simulink model "APE_Project_Closed Loop With Battery_SOC"  (R2025a)
settings: Solver=VariableStepAuto  StartTime=0.0  StopTime=0.05  RelTol=1e-3
undefined symbols (not defined in the file): Ion, Lithium
libraries: spsPWMGeneratorDCDCLib x8, spsCurrentMeasurementLib x5, spsMosfetLib x4, spsSeriesRLCBranchLib x4, spsVoltageMeasurementLib x3, spsBatteryLib x1, spsDCVoltageSourceLib x1, spsDiodeLib x1, spsGroundLib x1, eeStairGenerator x1, sps_lib x1
settings Model: Creator=KAILASH  LastModifiedBy=KAILASH

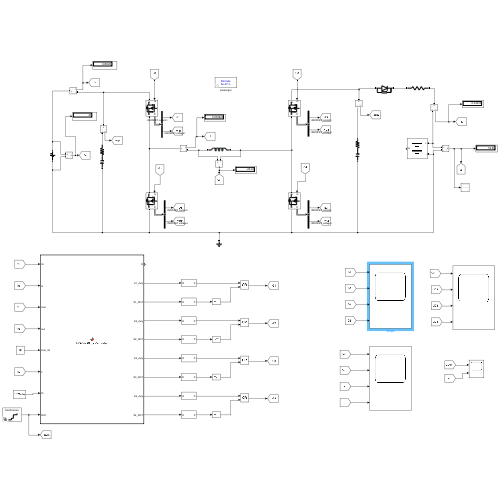
[thumbnail: Simulink's stored preview of the top-level diagram]
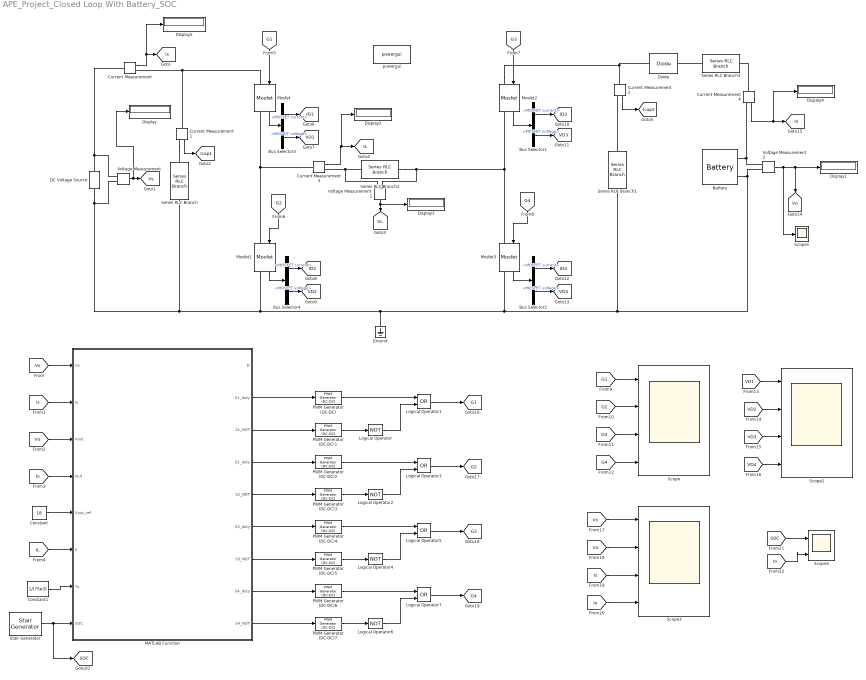
== system APE_Project_Closed Loop With Battery_SOC ==
  Battery : spsBatteryLib/Battery  BatType=Lithium-Ion  NomV=18  NomQ=5.4  SOC=95  Batt_Tr=30  PresetModel=on  MaxQ=5.4  MinV=13.5  FullV=20.9518  Dis_rate=2.3478  R=0.033333  Normal_OP=4.8835  expZone="[19.4469     0.265304]"
  Bus Selector{1..4} (4 alike) : BusSelector  OutputSignals=MOSFET current,MOSFET voltage
  Constant : Constant  Value=18
  Constant1 : Constant  Value=1/(75e3)
  Current Measurement{,1..4} (5 alike) : spsCurrentMeasurementLib/Current Measurement  PhasorSimulation=off  OutputType=Complex  PSBequivalent=0
  DC Voltage Source : spsDCVoltageSourceLib/DC Voltage Source  Amplitude=48  Measurements=Voltage
  Diode : spsDiodeLib/Diode  Ron=0.001  Lon=0  Vf=0.8  IC=0  UseSnubber=0  Rs=500  Cs=250e-9  Measurements=off
  Display{,1..5} (6 alike) : Display
  Ground : spsGroundLib/Ground  LConnTagsString=a
  Logical Operator{,2,4,6} (4 alike) : Logic  Operator=NOT  AllPortsSameDT=off  OutDataTypeStr=boolean
  Logical Operator{1,3,5,7} (4 alike) : Logic  Operator=OR  AllPortsSameDT=off  OutDataTypeStr=boolean
  MATLAB Function : MATLAB Function  TreatAsAtomicUnit=on
  Mosfet{,1..3} (4 alike) : spsMosfetLib/Mosfet  Ron=0.01  Lon=0  Rd=0.01  Vfd=0.8  IC=0  Rs=1e5  Cs=inf  Measurements=on
  PWM Generator (DC-DC){,1..7} (8 alike) : spsPWMGeneratorDCDCLib/PWM Generator (DC-DC)  Fsw=75e3  Ts=0
  Scope : Scope  NumInputPorts=4
      settings: ActiveDisplayYMinimum=-0.12499999999999997  ActiveDisplayYMaximum=1.125
  Scope1 : Scope
      settings: ActiveDisplayYMinimum=-2.5104550941550139  ActiveDisplayYMaximum=22.594095847395128
  Scope2 : Scope  NumInputPorts=4
      settings: ActiveDisplayYMinimum=-4.0101855999563254  ActiveDisplayYMaximum=36.044750018114769  DataLoggingVariableName=ScopeData2
  Scope3 : Scope  NumInputPorts=4
      settings: ActiveDisplayYMinimum=38  ActiveDisplayYMaximum=58  DataLoggingVariableName=ScopeData3
  Scope4 : Scope  NumInputPorts=2
      settings: ActiveDisplayYMinimum=10.625000000000002  ActiveDisplayYMaximum=104.375  DataLoggingVariableName=ScopeData4
  Series RLC Branch : spsSeriesRLCBranchLib/Series RLC Branch  LConnTagsString=__new0  RConnTagsString=__new0  BranchType=RC  Resistance=0.001  Inductance=1e-3  SetiL0=off  InitialCurrent=0  Capacitance=488e-6  Setx0=off  InitialVoltage=48  Measurements=None
  Series RLC Branch1 : spsSeriesRLCBranchLib/Series RLC Branch  LConnTagsString=__new0  RConnTagsString=__new0  BranchType=RC  Resistance=0.01  Inductance=1e-3  SetiL0=off  InitialCurrent=0  Capacitance=488e-6  Setx0=off  InitialVoltage=36  Measurements=None
  Series RLC Branch2 : spsSeriesRLCBranchLib/Series RLC Branch  LConnTagsString=__new0  RConnTagsString=__new0  BranchType=L  Resistance=1  Inductance=150e-6  SetiL0=off  InitialCurrent=0  Capacitance=1e-6  Setx0=off  InitialVoltage=0  Measurements=None
  Series RLC Branch3 : spsSeriesRLCBranchLib/Series RLC Branch  LConnTagsString=__new0  RConnTagsString=__new0  BranchType=R  Resistance=1  Inductance=1e-3  SetiL0=off  InitialCurrent=0  Capacitance=1e-6  Setx0=off  InitialVoltage=0  Measurements=None
  Stair Generator : eeStairGenerator/Stair Generator  LabelModeActiveChoice=Continuous  TimeInput=[0 0.02 0.03 0.05]  AmplitudeInput="[20  40 80 95]"  SampleTime=0  RepeatPattern=off  OutDataTypeStr=double
      settings: LibrarySourceBlock=ee_sl_lib/General Control/Stair Generator
  Voltage Measurement : spsVoltageMeasurementLib/Voltage Measurement  PhasorSimulation=off  OutputType=Complex  PSBequivalent=0
  Voltage Measurement1 : spsVoltageMeasurementLib/Voltage Measurement  PhasorSimulation=off  OutputType=Complex  PSBequivalent=0
  Voltage Measurement2 : spsVoltageMeasurementLib/Voltage Measurement  PhasorSimulation=off  OutputType=Complex  PSBequivalent=0
  powergui : sps_lib/powergui  Priority=1  SimulationMode=Discrete  SampleTime=5e-7  frequency=60  Iterations=50  frequencyindice=0  Pbase=100e6  ErrMax=1e-4  UnitsV=kV  UnitsW=MW  buscounter=0  FunctionMessages=off  echomessages=off  EnableUseOfTLC=off  CurrentSourceSwitches=off  DisableSnubberDevices=off  DisableRonSwitches=off  DisableVfSwitches=off  DisplayEquations=off  AutomaticDiscreteSolvers=off  SolverType=Tustin/Backward Euler (TBE)  Interpol=off  ExternalGateDelay=off  methode=off  Ts=100  x0status=blocks  SPID=on  SwTol=0  HookPort=off  NonlinearTolerance=1e-4  nMaxIteration=100  ContinueOnMaxIteration=off  RestoreLinks=warning  ResistiveCurrentMeasurement=off  Frange=[0:2:500]  Ylog=off  Xlog=on  ShowGrid=off  save=off  variable=ZData  structure=0  ZoomFFT=off  StartTime=0.0  cycles=1  DisplayStyle=1  fundamental=60  FreqAxis=off  MaxFrequency=1000  frequencyindicesteady=1  RmsSteady=1  display=off
  tag scope: G1=global, G2=global, G3=global, G4=global, ID1=global, ID2=global, ID3=global, ID4=global, IL=global, Icap1=global, Icap2=global, Io=global, Is=global, SOC=global, VD1=global, VD2=global, VD3=global, VD4=global, VL=global, Vo=global, Vs=global
  wires:
  [G4] -> Mosfet3/1
  Logical Operator3/1 -> [G2]
  [G3] -> Scope/3
  [G1] -> Mosfet/1
  Logical Operator5/1 -> [G3]
  Constant/1 -> MATLAB Function/5(Vout_ref)
  [Vo] -> MATLAB Function/3(Vout)
  MATLAB Function/7(S3_NOT) -> PWM Generator (DC-DC)5/1
  Logical Operator2/1 -> Logical Operator3/2
  PWM Generator (DC-DC)2/1 -> Logical Operator3/1
  PWM Generator (DC-DC)3/1 -> Logical Operator2/1
  [G2] -> Mosfet1/1
  PWM Generator (DC-DC)6/1 -> Logical Operator7/1
  Logical Operator6/1 -> Logical Operator7/2
  [Vs] -> MATLAB Function/1(Vs)
  PWM Generator (DC-DC)7/1 -> Logical Operator6/1
  Logical Operator4/1 -> Logical Operator5/2
  [G1] -> Scope/1
  [G3] -> Mosfet2/1
  [Vo] -> Scope3/2
  Constant1/1 -> MATLAB Function/7(Ts)
  MATLAB Function/6(S3_duty) -> PWM Generator (DC-DC)4/1
  Logical Operator/1 -> Logical Operator1/2
  PWM Generator (DC-DC)1/1 -> Logical Operator/1
  [Is] -> MATLAB Function/2(Is)
  MATLAB Function/8(S4_duty) -> PWM Generator (DC-DC)6/1
  PWM Generator (DC-DC)/1 -> Logical Operator1/1
  Bus Selector1/2 -> [VD3]  "<MOSFET voltage>"
  Current Measurement3/1 -> Display2/1, [IL]
  Current Measurement2/1 -> [Icap2]
  [G2] -> Scope/2
  Bus Selector3/2 -> [VD1]  "<MOSFET voltage>"
  [VD2] -> Scope2/2
  Mosfet1/1 -> Bus Selector4/1
  Bus Selector4/2 -> [VD2]  "<MOSFET voltage>"
  Mosfet/1 -> Bus Selector3/1
  Voltage Measurement1/1 -> Display3/1, [VL]
  Mosfet2/1 -> Bus Selector1/1
  Bus Selector4/1 -> [ID2]  "<MOSFET current>"
  Bus Selector3/1 -> [ID1]  "<MOSFET current>"
  Voltage Measurement/1 -> Display/1, [Vs]
  PWM Generator (DC-DC)4/1 -> Logical Operator5/1
  Logical Operator1/1 -> [G1]
  Current Measurement4/1 -> Display4/1, [Io]
  Voltage Measurement2/1 -> Scope1/1, [Vo], Display1/1
  [VD1] -> Scope2/1
  [VD3] -> Scope2/3
  Current Measurement/1 -> Display5/1, [Is]
  Mosfet3/1 -> Bus Selector2/1
  [IL] -> MATLAB Function/6(Il)
  Logical Operator7/1 -> [G4]
  Bus Selector2/2 -> [VD4]  "<MOSFET voltage>"
  [VD4] -> Scope2/4
  MATLAB Function/5(S2_NOT) -> PWM Generator (DC-DC)3/1
  Bus Selector2/1 -> [ID4]  "<MOSFET current>"
  MATLAB Function/9(S4_NOT) -> PWM Generator (DC-DC)7/1
  [Io] -> Scope3/4
  [Vs] -> Scope3/1
  [G4] -> Scope/4
  [Is] -> Scope3/3
  [Io] -> MATLAB Function/4(Iout)
  PWM Generator (DC-DC)5/1 -> Logical Operator4/1
  Current Measurement1/1 -> [Icap1]
  MATLAB Function/2(S1_duty) -> PWM Generator (DC-DC)/1
  Bus Selector1/1 -> [ID3]  "<MOSFET current>"
  MATLAB Function/4(S2_duty) -> PWM Generator (DC-DC)2/1
  MATLAB Function/3(S1_NOT) -> PWM Generator (DC-DC)1/1
  Stair Generator/1 -> [SOC], MATLAB Function/8(SOC)
  [SOC] -> Scope4/1
  [Io] -> Scope4/2
  connections:
  Mosfet3/LConn1 -- Mosfet2/RConn1 -- Voltage Measurement1/LConn2 -- Series RLC Branch2/RConn1
  Battery/LConn2 -- Voltage Measurement2/LConn2 -- Series RLC Branch1/RConn1 -- Ground/LConn1 -- Mosfet1/RConn1 -- Series RLC Branch/RConn1 -- Voltage Measurement/LConn2 -- DC Voltage Source/LConn1 -- Mosfet3/RConn1
  Mosfet2/LConn1 -- Current Measurement2/LConn1 -- Diode/LConn1
  Voltage Measurement1/LConn1 -- Current Measurement3/RConn1 -- Series RLC Branch2/LConn1
  Battery/LConn1 -- Current Measurement4/RConn1 -- Voltage Measurement2/LConn1
  Voltage Measurement/LConn1 -- Current Measurement/LConn1 -- DC Voltage Source/RConn1
  Current Measurement3/LConn1 -- Mosfet/RConn1 -- Mosfet1/LConn1
  Current Measurement1/LConn1 -- Current Measurement/RConn1 -- Mosfet/LConn1
  Series RLC Branch3/LConn1 -- Diode/RConn1
  Series RLC Branch1/LConn1 -- Current Measurement2/RConn1
  Current Measurement1/RConn1 -- Series RLC Branch/LConn1
  Current Measurement4/LConn1 -- Series RLC Branch3/RConn1

== matlab function APE_Project_Closed Loop With Battery_SOC/MATLAB Function ==
  data: Vs input; D output; Is input; Vout input; Iout input; Vout_ref input; Il input; Ts input; S1_duty output; S1_NOT output; S2_duty output; S2_NOT output; S3_duty output; S3_NOT output; S4_duty output; S4_NOT output; SOC input
function [D, S1_duty, S1_NOT, S2_duty, S2_NOT, S3_duty, S3_NOT, S4_duty, S4_NOT] = biDirBuckBoostController(Vs, Is, Vout, Iout, Vout_ref, Il, Ts, SOC)
% Bidirectional 4-switch DC-DC controller 
% Auto-Mode Detection with Noise-Immune Hysteresis (Deadband)
% Charge Mode: Hybrid SOC Profile + CV Safety Limit
% Discharge Mode: Cascaded Voltage/Current loop with Feedforward
% %#codegen

%% ===================== GLOBAL VARIABLES =====================
% Safety / clamping
D_MAX = 0.92;
D_MIN = 0.1;
V_HYST_CHRG = 4.5; % hysteresis band (V) for topology switching

%% ===================== CHARGING VARIABLES =====================
persistent v_int_chg i_int_chg
if isempty(v_int_chg), v_int_chg = 0; end
if isempty(i_int_chg), i_int_chg = 0; end

% SOC Profile Settings
I_MAX_BULK = 5.0;       % Max current during 0-80% (A)
I_MIN_TAPER = 0.5;      % End-of-charge current at 99% (A)
SOC_BULK_END = 80.0;    % When to start tapering current (%)
SOC_FULL = 100.0;       % When to stop charging completely (%)

% Gains
Kp_v_chg = 0.5;        Ki_v_chg = 15.0;  % Outer CV loop gains (Safety Brake)
Kp_i_chg = 0.05;       Ki_i_chg = 40.0;  % Inner CC loop gains (Muscle)

%% ===================== DISCHARGE VARIABLES =====================
persistent v_int_dis i_int_dis R_est_prev
if isempty(v_int_dis), v_int_dis = 0; end
if isempty(i_int_dis), i_int_dis = 0; end
if isempty(R_est_prev), R_est_prev = 3; end

%% ===================== INITIALIZE OUTPUTS =====================
D = 0.0;
S1_duty = 0.0; S1_NOT  = 1.0;
S2_duty = 0.0; S2_NOT  = 1.0;
S3_duty = 0.0; S3_NOT  = 1.0;
S4_duty = 0.0; S4_NOT  = 1.0;

%% ===================== AUTO MODE DETECTION (DEADBAND) =====================
persistent is_charging_state
if isempty(is_charging_state)
    is_charging_state = true; % Default startup state
end

% The Noise Immunity Band (Amps)
I_DEADBAND = 0.1; 
if is_charging_state == true
    if Il < -I_DEADBAND
        is_charging_state = false;
    end
else
    if Il > I_DEADBAND
        is_charging_state = true;
    end
end
is_charging = is_charging_state;

%% ===================== CHARGE MODE CONTROL (HYBRID SOC) =====================
if is_charging
    
    % --- 1. SOC PROFILE MANAGER ---
    if SOC < SOC_BULK_END
        I_soc_limit = I_MAX_BULK;
    elseif SOC >= SOC_FULL
        I_soc_limit = 0.0;
    else
        % Linear taper down as battery approaches 100%
        fraction = (SOC - SOC_BULK_END) / (SOC_FULL - SOC_BULK_END);
        I_soc_limit = I_MAX_BULK - (fraction * (I_MAX_BULK - I_MIN_TAPER));
    end

    % --- 2. OUTER VOLTAGE LOOP (Safety Brake) ---
    v_err = Vout_ref - Vout;
    v_int_chg = v_int_chg + Ki_v_chg * v_err * Ts;
    
    % Anti-windup: Clamp to the dynamic SOC limit instead of a fixed 5.0A
    v_int_chg = min(max(v_int_chg, 0.0), I_soc_limit);
    
    % Calculate requested current and clamp to dynamic SOC limit
    I_target = Kp_v_chg * v_err + v_int_chg;
    I_target = min(max(I_target, 0.0), I_soc_limit);
    
    % --- 3. INNER CURRENT LOOP ---
    i_err = I_target - Iout;
    i_int_chg = i_int_chg + Ki_i_chg * i_err * Ts;
    i_int_chg = min(max(i_int_chg, D_MIN), D_MAX);
    D_unsat = Kp_i_chg * i_err + i_int_chg;
    
    % Final Saturation & Anti-windup
    if D_unsat > D_MAX
        D = D_MAX;
        i_int_chg = i_int_chg - Ki_i_chg * i_err * Ts;
    elseif D_unsat < D_MIN
        D = D_MIN;
        i_int_chg = i_int_chg - Ki_i_chg * i_err * Ts;
    else
        D = D_unsat;
    end

    % --- SWITCH MAPPING (TOPOLOGY SELECTOR) ---
    if Vs > Vout - V_HYST_CHRG && Vs < Vout + V_HYST_CHRG
        % Buck-boost region
        S1_duty = D;      S1_NOT  = 1.0;
        S2_duty = 0.0;    S2_NOT  = D;
        S3_duty = 0.0;    S3_NOT  = D;
        S4_duty = D;      S4_NOT  = 1.0;
    elseif Vs > Vout + V_HYST_CHRG
        % Buck region
        S1_duty = D;      S1_NOT  = 1.0;
        S2_duty = 0.0;    S2_NOT  = D;
        S3_duty = 1.0;    S3_NOT  = 1.0;
        S4_duty = 0.0;    S4_NOT  = 1.0;
    else
        % Boost region 
        S1_duty = 1.0;    S1_NOT  = 1.0;
        S2_duty = 0.0;    S2_NOT  = 1.0;
        S3_duty = 0.0;    S3_NOT  = D;
        S4_duty = D;      S4_NOT  = 1.0;
    end
    return;

%% ===================== DISCHARGE MODE CONTROL =====================
else
    % ----- Reference & limits -----
    Vref_led      = 14.4;        
    V_HYST_DISCH  = 0.50;        
    I_target_nom  = 1.0;         
    I_abs_max     = 1.4;         
    I_HYST_DISCH  = 0.01;        

    % ----- Gains -----
    Kp_v = 0.12;   Ki_v = 40;   
    Kp_i = 0.45;   Ki_i = 270;  
    FF_mix = 0.6;               

    % ----- Measured variables -----
    I_load = -Is;               
    V_load = Vs;                
    V_batt = Vout;              

    % ================= OUTER VOLTAGE LOOP =================
    v_err = Vref_led - V_load;
    if abs(v_err) > V_HYST_DISCH
        v_int_dis = v_int_dis + Ki_v * v_err * Ts;
    end
    v_int_dis = min(max(v_int_dis, -1.0), 1.0);
    I_target = Kp_v * v_err + v_int_dis + I_target_nom;
    I_target = min(max(I_target, 0.0), I_abs_max);

    % ================= INNER CURRENT LOOP & FEEDFORWARD =================
    epsI = 1e-4;
    R_inst = V_load / max(I_load, epsI);
    alphaR = 0.08;
    R_est = (1 - alphaR) * R_est_prev + alphaR * R_inst;
    R_est_prev = R_est;
    V_load_ff = I_target * R_est;
    if V_load_ff <= V_batt
        D_ff = V_load_ff / max(V_batt, 1e-6);      % buck
    else
        D_ff = 1 - (V_batt / max(V_load_ff, 1e-6)); % boost
    end
    D_ff = min(max(D_ff, D_MIN), D_MAX);

    % Current PI
    i_err = I_target - I_load;
    if abs(i_err) > I_HYST_DISCH
        i_int_dis = i_int_dis + Ki_i * i_err * Ts;
    end
    i_int_dis = min(max(i_int_dis, -0.6), 0.6);
    D_corr = Kp_i * i_err + i_int_dis;

    % Combine FF + correction 
    D_unsat = FF_mix * D_ff + (1 - FF_mix) * (D_ff + D_corr);
    if D_unsat > D_MAX
        D = D_MAX;
        i_int_dis = i_int_dis - Ki_i * i_err * Ts;
    elseif D_unsat < D_MIN
        D = D_MIN;
        i_int_dis = i_int_dis - Ki_i * i_err * Ts;
    else
        D = D_unsat;
    end
    if I_load > (I_abs_max + I_HYST_DISCH)
        D = max(D_MIN, D * 0.5);
        i_int_dis = 0;
    end

    % ================= SWITCH MAPPING =================
    if Vs > Vout + V_HYST_CHRG
        S1_duty = 0;  S1_NOT = D;
        S2_duty = D;  S2_NOT = 1;
        S3_duty = 1;  S3_NOT = 1;
        S4_duty = 0;  S4_NOT = 1;
    elseif Vs < Vout - V_HYST_CHRG
        S1_duty = 1;  S1_NOT = 1;
        S2_duty = 0;  S2_NOT = 1;
        S3_duty = D;  S3_NOT = 1;
        S4_duty = 0;  S4_NOT = D;
    else
        S1_duty = 0;  S1_NOT = D;
        S2_duty = D;  S2_NOT = 1;
        S3_duty = D;  S3_NOT = 1;
        S4_duty = 0;  S4_NOT = D;
    end
    return;
end

%% ===================== DEFAULT / SAFE OUTPUTS =====================
D = 0.0;
S1_duty = 0.0; S1_NOT  = 1.0;
S2_duty = 0.0; S2_NOT  = 1.0;
S3_duty = 0.0; S3_NOT  = 1.0;
S4_duty = 0.0; S4_NOT  = 1.0;
end
